simulink model "Position_System_saturation_control101"  (R2023a)
settings: Solver=ode45  StartTime=0.0  StopTime=2.0  RelTol=1e-3  EnableMultiTasking=on
values from neighbouring files (symbols this model uses):
  C = 6000    [simulink_openloop_model_control101_script.m]    (also in simulink_openloop_modelb_control101_script.m; simulink_openloop_modelc_control101_script.m = 2000; simulink_openloop_modeld_control101_script.m = 1000)
undefined symbols (not defined in the file or in its folder): d, km, ks, P, R
settings Model: Creator=stelios  LastModifiedBy=Anthony Rossiter
settings DataIOCC: LimitDataPoints=on  SaveFormat=Array  SignalLoggingSaveFormat=ModelDataLogs  ReturnWorkspaceOutputs=off
settings OptimizationCC: BooleanDataType=off
settings DebuggingCC: SaveWithParameterizedLinksMsg=none  UnderspecifiedInitializationDetection=Classic  MergeDetectMultiDrivingBlocksExec=none  SignalResolutionControl=TryResolveAllWithWarning  InheritedTsInSrcMsg=none  MultiTaskDSMMsg=warning  MultiTaskCondExecSysMsg=none  UnconnectedInputMsg=warning  UnconnectedOutputMsg=warning  UnconnectedLineMsg=warning
settings HardwareCC: TargetUnknown=on
settings ModelReferenceCC: EnableRefExpFcnMdlSchedulingChecks=on  PropagateSignalLabelsOutOfModel=off
settings RTWCC: DLArmComputeVersion=19.05
settings GRTTargetCC: CombineOutputUpdateFcns=off  GRTInterface=on
settings ConfigComp: CovMetricSettings=dw

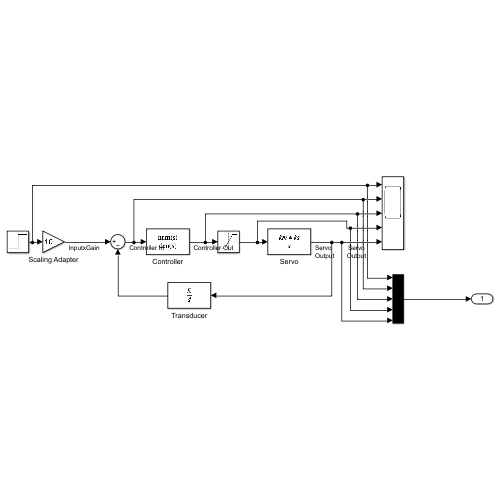
[thumbnail: Simulink's stored preview of the top-level diagram]
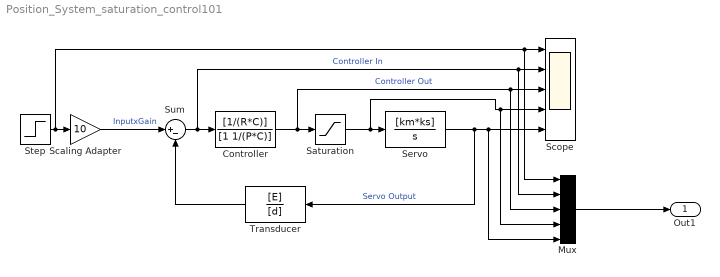
== system Position_System_saturation_control101 ==
  Controller : TransferFcn  Numerator=[1/(R*C)]  Denominator=[1 1/(P*C)]
  Mux : Mux  Inputs=5
  Saturation : Saturate  UpperLimit=10  LowerLimit=-10
  Scaling Adapter : Gain  Gain=10  SaturateOnIntegerOverflow=on
  Scope : Scope  NumInputPorts=5
  Servo : TransferFcn  Numerator=[km*ks]  Denominator=[1 0]
  Step : Step  After=1.3
  Sum : Sum  Inputs=|+-  SaturateOnIntegerOverflow=on
  Transducer : TransferFcn  Numerator=[E]  Denominator=[d]
  Out1 : Outport
  wires:
  Sum/1 -> Mux/2, Scope/2, Controller/1  "Controller In"
  Servo/1 -> Transducer/1, Mux/5, Scope/5  "Servo Output"
  Transducer/1 -> Sum/2
  Step/1 -> Mux/1, Scope/1, Scaling Adapter/1
  Scaling Adapter/1 -> Sum/1  "InputxGain"
  Saturation/1 -> Mux/4, Scope/4, Servo/1
  Controller/1 -> Mux/3, Scope/3, Saturation/1  "Controller Out"
  Mux/1 -> Out1/1
